simulink model "SPHERE_model4"  (R2020a)
settings: Solver=ode4  StartTime=0.0  StopTime=35  FixedStep=0.01428571  RelTol=1e-3
values from neighbouring files (symbols this model uses):
  Final_val = 18    [Initial_script.m]    (also in Initial_script_test.m = -28; Initial_script_test2.m = -28)
  K = 25.937    [Initial_script.m]    (also in Initial_script_test.m; Initial_script_test2.m)
  L = -[ M2*l*(-2*l + R) - 2*J2, 0, -2*M2*l*g ]    [Initial_script.m]    (also in Initial_script_test.m; Initial_script_test2.m)
  M = [ J1 + 2*J2 + M1*R^2 + M2*(2*l^2 - 3*R*l + R^2), -Tv, 2*l*g*M2 ]    [Initial_script.m]    (also in Initial_script_test.m; Initial_script_test2.m)
  Smax = 502    [Initial_script.m]    (also in Initial_script_test.m; Initial_script_test2.m)
  Smin = -480    [Initial_script.m]    (also in Initial_script_test.m; Initial_script_test2.m)
  Step_time = 3.18    [Initial_script.m]    (also in Initial_script_test.m = 4.45; Initial_script_test2.m = 4.5)
  Top = 0.015    [Initial_script.m]    (also in Initial_script_test.m; Initial_script_test2.m)
settings Model: Creator=Adrian  LastModifiedBy=Adrian

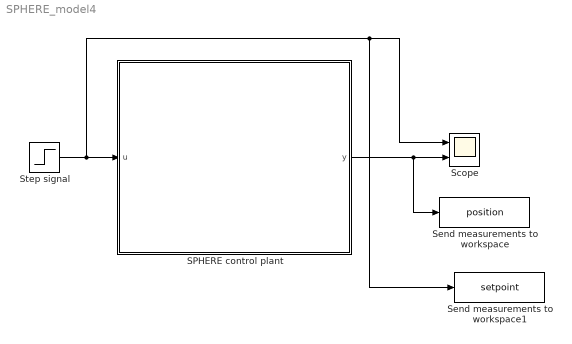
== system SPHERE_model4 ==
  SPHERE control plant : Subsystem
      mask Display: image('C:\Users\Adrian\Documents\Praca Magisterska\Robot kulisty by Adrian\Praca Magisterska\LaTex\Pictures\Old\sphere_full.PNG'); % Use "Edit Image" on toolstrip to change.
  Scope : Scope  NumInputPorts=2
  Send measurements to workspace : ToWorkspace  VariableName=position  SaveFormat=Timeseries  SampleTime=-1
  Send measurements to workspace1 : ToWorkspace  VariableName=setpoint  SaveFormat=Timeseries  SampleTime=-1
  Step signal : Step  Time=Step_time  After=Final_val  SampleTime=0
  wires:
  Step signal/1 -> Send measurements to workspace1/1, Scope/1, SPHERE control plant/1(u)
  SPHERE control plant/1(y) -> Send measurements to workspace/1, Scope/2

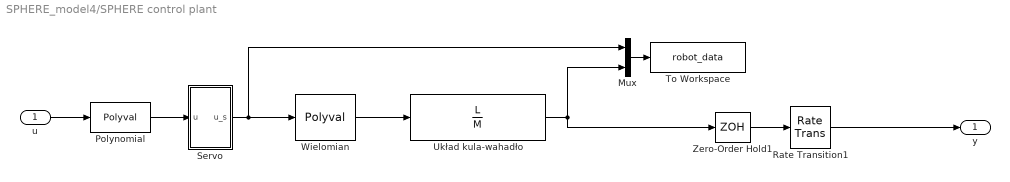
== system SPHERE_model4/SPHERE control plant ==
  u : Inport
  Mux : Mux  Inputs=2
  Polynomial : Polyval  Coefs=[0.000325 0.001274 1.044515 0]
  Rate Transition1 : RateTransition
  Servo : Subsystem
  To Workspace : ToWorkspace  VariableName=robot_data  SaveFormat=Structure With Time  SampleTime=-1
  Układ kula-wahadło : TransferFcn  Numerator=L  Denominator=M
  Wielomian : Polyval  Coefs=[-0.000067 -0.000287 0.871698 0]
  Zero-Order Hold1 : ZeroOrderHold  SampleTime=-1
  y : Outport
  wires:
  u/1 -> Polynomial/1
  Układ kula-wahadło/1 -> Mux/2, Zero-Order Hold1/1
  Servo/1(u_s) -> Wielomian/1, Mux/1
  Mux/1 -> To Workspace/1
  Zero-Order Hold1/1 -> Rate Transition1/1
  Rate Transition1/1 -> y/1
  Wielomian/1 -> Układ kula-wahadło/1
  Polynomial/1 -> Servo/1(u)

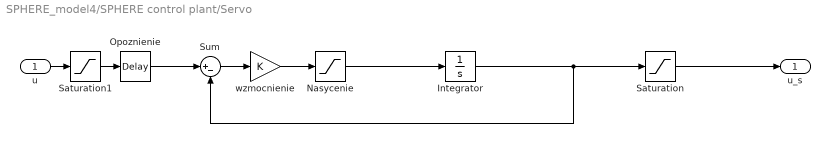
== system SPHERE_model4/SPHERE control plant/Servo ==
  u : Inport
  Integrator : Integrator
  Nasycenie : Saturate  UpperLimit=Smax  LowerLimit=Smin
  Opoznienie : TransportDelay  DelayTime=Top
  Saturation : Saturate  UpperLimit=60  LowerLimit=-60
  Saturation1 : Saturate  UpperLimit=60  LowerLimit=-60
  Sum : Sum  Inputs=|+-
  wzmocnienie : Gain  Gain=K
  u_s : Outport
  wires:
  Sum/1 -> wzmocnienie/1
  Integrator/1 -> Saturation/1, Sum/2
  wzmocnienie/1 -> Nasycenie/1
  Opoznienie/1 -> Sum/1
  Nasycenie/1 -> Integrator/1
  u/1 -> Saturation1/1
  Saturation/1 -> u_s/1
  Saturation1/1 -> Opoznienie/1
